simulink model "absSimulation"  (R2013b)
settings: Solver=ode3  StartTime=0.0  StopTime=60  FixedStep=0.0001  MaxStep=0.01  RelTol=1e-3
InitFcn:
  | initAbsSim
StartFcn:
  | initAbsSim
values from neighbouring files (symbols this model uses):
  g = 9.81    [abssim1.mat]    (also in abssim2.mat; abssim3.mat; initAbsSim.m)
  m = 9    [abssim1.mat]    (also in abssim2.mat; abssim3.mat; initAbsSim.m)
  Rd = 0.0625    [abssim1.mat]    (also in abssim2.mat; abssim3.mat; initAbsSim.m)
  tyreData = [0 0.0585778811244 0.114421508325 0.16758915878 0.218139109665 0.266129638158 0.311619021435 0.354665536675 0.395327461053 0.433663071746 0.469730645933 0.503588460789 ... (101 elements, 1x101)]    [abssim1.mat]    (also in abssim2.mat; abssim3.mat; tyreDataGen.m = interp1(x,v,xq, 'spline'))
  v0 = 20    [abssim1.mat]    (also in abssim2.mat; abssim3.mat; initAbsSim.m = 5)
libraries: simulink x2
settings Model: FPTRunName=FPA_Reference  Creator=lasse  LastModifiedBy=Lasse
settings DebuggingCC: SignalRangeChecking=warning
settings HardwareCC: ProdBitPerInt=16  ProdBitPerPointer=8  ProdIntDivRoundTo=Zero  ProdEndianess=LittleEndian  ProdWordSize=8  ProdHWDeviceType=Atmel->AVR
settings ModelReferenceCC: ModelReferenceMinAlgLoopOccurrences=on

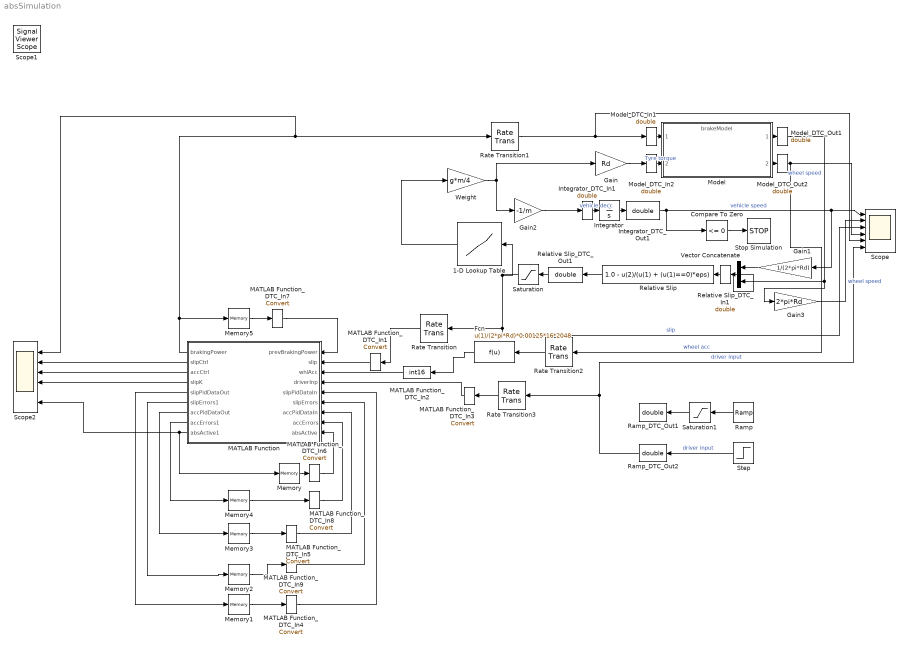
== system absSimulation ==
  1-D Lookup Table : Lookup_n-D  NumberOfTableDimensions=1  BreakpointsForDimension1=[0:100]  Table=tyreData(1:101)  TableDataTypeStr=double  OutDataTypeStr=double  RndMeth=Simplest  InputSameDT=on
  Compare To Zero : simulink/Logic and Bit Operations/Compare To Zero  relop=<=  OutDataTypeStr=boolean
  Fcn : Fcn  Expr=u(1)/(2*pi*Rd)*0.00125*16*2048
  Gain : Gain  Gain=Rd  OutDataTypeStr=double
  Gain1 : Gain  Gain=1/(2*pi*Rd)  OutDataTypeStr=double
  Gain2 : Gain  Gain=-1/m  OutDataTypeStr=double
  Gain3 : Gain  Gain=2*pi*Rd  OutDataTypeStr=double
  Integrator : Integrator  InitialCondition=v0
  Integrator_DTC_In1 : DataTypeConversion  Tag=InsertedToIsolateUnsupportedBlock  OutDataTypeStr=double  LockScale=on
  Integrator_DTC_Out1 : DataTypeConversion  OutDataTypeStr=double
  MATLAB Function : MATLAB Function  TreatAsAtomicUnit=on  SystemSampleTime=0.01
  MATLAB Function_DTC_In{1,3..9} (8 alike) : DataTypeConversion
  MATLAB Function_DTC_In2 : DataTypeConversion  Tag=InsertedToIsolateUnsupportedBlock  OutDataTypeStr=int16  LockScale=on
  Memory : Memory  InheritSampleTime=on
  Memory1 : Memory  X0="[128  100 0 100 0]*2^8"  InheritSampleTime=on
  Memory2 : Memory  X0=[0 0]  InheritSampleTime=on
  Memory3 : Memory  X0=[5 1 0 0 100 0]*2^8  InheritSampleTime=on
  Memory4 : Memory  X0=[0 0]  InheritSampleTime=on
  Memory5 : Memory  InheritSampleTime=on
  Model : ModelReference  ModelNameDialog=brakeModel.slx  SimulationMode=Normal  ModelReferenceVersion=1.18  CopyOfModelName=brakeModel.slx  DefaultDataLogging=on
  Model_DTC_In1 : DataTypeConversion  Tag=InsertedToIsolateUnsupportedBlock  OutDataTypeStr=double  LockScale=on
  Model_DTC_In2 : DataTypeConversion  Tag=InsertedToIsolateUnsupportedBlock  OutDataTypeStr=double  LockScale=on
  Model_DTC_Out1 : DataTypeConversion  OutDataTypeStr=double
  Model_DTC_Out2 : DataTypeConversion  OutDataTypeStr=double
  Ramp : simulink/Sources/Ramp  slope=10  start=0  X0=0
  Ramp_DTC_Out1 : DataTypeConversion  OutDataTypeStr=double
  Ramp_DTC_Out2 : DataTypeConversion  OutDataTypeStr=double
  Rate Transition : RateTransition  OutPortSampleTime=0.01
  Rate Transition1 : RateTransition  OutPortSampleTimeOpt=Inherit  OutPortSampleTime=0.01
  Rate Transition2 : RateTransition  OutPortSampleTime=0.01
  Rate Transition3 : RateTransition  OutPortSampleTime=0.01
  Relative Slip : Fcn  Expr=1.0 - u(2)/(u(1) + (u(1)==0)*eps)
  Relative Slip_DTC_In1 : DataTypeConversion  Tag=InsertedToIsolateUnsupportedBlock  OutDataTypeStr=double  LockScale=on
  Relative Slip_DTC_Out1 : DataTypeConversion  OutDataTypeStr=double
  Saturation : Saturate  UpperLimit=1.0  LowerLimit=0  OutDataTypeStr=double
  Saturation1 : Saturate  UpperLimit=500  LowerLimit=0
  Scope : Scope  NumInputPorts=6
      settings: YMin=19.9955~19.1~0~-17.5~0~475  YMax=20~20~0.045~5~100~525
  Scope2 : Scope  NumInputPorts=6
      settings: YMin=0~19000~-35000~0~-1~0  YMax=100~33000~35000~100~1~1
  Step : Step  After=500  SampleTime=0
  Stop Simulation : Stop
  Vector Concatenate : Concatenate
  Weight : Gain  Gain=g*m/4  OutDataTypeStr=double
  Scope1 : SignalViewerScope  IOType=viewer  RefreshTime=0.035000
  wires:
  Model/1 -> Model_DTC_Out1/1
  Gain1/1 -> Vector Concatenate/1
  Vector Concatenate/1 -> Relative Slip_DTC_In1/1
  Relative Slip/1 -> Relative Slip_DTC_Out1/1
  Weight/1 -> Gain2/1, Gain/1
  Gain/1 -> Model_DTC_In2/1
  Gain2/1 -> Integrator_DTC_In1/1
  Integrator/1 -> Integrator_DTC_Out1/1
  Compare To Zero/1 -> Stop Simulation/1
  Saturation/1 -> Rate Transition/1, Scope/3, 1-D Lookup Table/1  "slip"
  Gain3/1 -> Scope/2  "wheel speed"
  Model/2 -> Model_DTC_Out2/1
  Ramp/1 -> Saturation1/1
  Rate Transition1/1 -> Model_DTC_In1/1, Scope/5
  1-D Lookup Table/1 -> Weight/1
  Ramp_DTC_Out2/1 -> Scope/6, Rate Transition3/1  "driver input"
  Integrator_DTC_Out1/1 -> Scope/1, Gain1/1, Compare To Zero/1  "vehicle speed"
  Relative Slip_DTC_Out1/1 -> Saturation/1
  Relative Slip_DTC_In1/1 -> Relative Slip/1
  Model_DTC_In1/1 -> Model/1
  Model_DTC_In2/1 -> Model/2  "Tyre torque"
  Model_DTC_Out1/1 -> Gain3/1, Vector Concatenate/2  "wheel speed"
  Model_DTC_Out2/1 -> Scope/4, Rate Transition2/1  "wheel acc"
  Rate Transition/1 -> MATLAB Function_DTC_In1/1
  Integrator_DTC_In1/1 -> Integrator/1  "vehicle decc"
  Step/1 -> Ramp_DTC_Out2/1  "driver input"
  Rate Transition2/1 -> Fcn/1
  Fcn/1 -> MATLAB Function_DTC_In2/1
  MATLAB Function_DTC_In2/1 -> MATLAB Function/3(whlAcc)
  Rate Transition3/1 -> MATLAB Function_DTC_In3/1
  MATLAB Function/7(accPidDataOut) -> Memory3/1
  MATLAB Function/9(absActive1) -> Memory/1, Scope2/6
  Memory1/1 -> MATLAB Function_DTC_In4/1
  Memory3/1 -> MATLAB Function_DTC_In5/1
  Memory/1 -> MATLAB Function_DTC_In6/1
  MATLAB Function/2(slipCtrl) -> Scope2/2
  MATLAB Function/3(accCtrl) -> Scope2/3
  MATLAB Function/4(slipK) -> Scope2/4
  MATLAB Function_DTC_In1/1 -> MATLAB Function/2(slip)
  MATLAB Function_DTC_In3/1 -> MATLAB Function/4(driverInp)
  MATLAB Function_DTC_In4/1 -> MATLAB Function/5(slipPidDataIn)
  MATLAB Function_DTC_In5/1 -> MATLAB Function/7(accPidDataIn)
  MATLAB Function_DTC_In6/1 -> MATLAB Function/9(absActive)
  Saturation1/1 -> Ramp_DTC_Out1/1
  MATLAB Function/5(slipPidDataOut) -> Memory1/1
  MATLAB Function/8(accErrors1) -> Memory4/1
  Memory4/1 -> MATLAB Function_DTC_In8/1
  MATLAB Function/6(slipErrors1) -> Memory2/1
  Memory2/1 -> MATLAB Function_DTC_In9/1
  MATLAB Function_DTC_In7/1 -> MATLAB Function/1(prevBrakingPower)
  MATLAB Function_DTC_In8/1 -> MATLAB Function/8(accErrors)
  MATLAB Function_DTC_In9/1 -> MATLAB Function/6(slipErrors)
  Memory5/1 -> MATLAB Function_DTC_In7/1
  MATLAB Function/1(brakingPower) -> Scope2/1, Rate Transition1/1, Memory5/1

== matlab function absSimulation/MATLAB Function ==
  data: prevBrakingPower input; slip input; brakingPower output; slipCtrl output; accCtrl output; slipK output; slipPidDataOut output; slipErrors1 output; whlAcc input; driverInp input; slipPidDataIn input; slipErrors input; accPidDataOut output; accErrors1 output; accPidDataIn input; accErrors input; absActive input; absActive1 output
function [brakingPower, slipCtrl, accCtrl, slipK, slipPidDataOut, slipErrors1, accPidDataOut, accErrors1, absActive1]= fcn(prevBrakingPower, slip,whlAcc,driverInp, slipPidDataIn, slipErrors, accPidDataIn, accErrors, absActive)
% %%%%%%%%%
%     sampleT = 0.00125;
%     PPR = 2048;
%     Rd = 0.0625;
%     desiredSlip = int8(33);
%     
%     desiredAcc = -5;
%     desiredAccInt = int16(desiredAcc/(2*pi*Rd)*sampleT*16*PPR);
%     slipParamsPID = [20 10 0 0.01, prevBrakingPower];
%     accParamsPID = [1 0.5 0 0.01 prevBrakingPower];
%     
%     if abs(whlAcc) > 1000
%         slipK = int8(0);
%     elseif abs(whlAcc) < 10
%         slipK = int8(100);
%     else
%         slipK = int8(100) - int8(abs(whlAcc)/1000);
%     end
% 
%     [slipCtrl, eSlip] = PID(slip, desiredSlip, slipErrors, slipParamsPID);
%     [accCtrl, eAcc] = PID(-whlAcc, desiredAccInt, accErrors, accParamsPID);
% 
%     slipErrors1 = [eSlip slipErrors(1)];
%     accErrors1 = [eAcc accErrors(1)];
%     if absActive
%         brakingPower = prevBrakingPower + slipK*int8(slipCtrl) + (int8(100)-slipK)*int8(accCtrl);
%         absActive1 = absActive;
%     else
%         brakingPower = int8(driverInp);
%         if whlAcc < desiredAcc || slip > desiredSlip
%             absActive1 = 1;
%         else
%             absActive1 = 0;
%         end
%     end
%     
%     brakingPower = checkSaturation(brakingPower, int8([0 100])); 
% %%%    

    sampleT = 0.00125;
    PPR = 2048;
    Rd = 0.0625;
    desiredSlip = int16(33);
    slipPercent = int16(slip*100);
    desiredAcc = -5;
    desiredAccInt = int16(desiredAcc/(2*pi*Rd)*sampleT*16*PPR);
    slipPidData = int16(slipPidDataIn);
    [slipCtrl, slipPidDataOut] = PID(slipPidData, desiredSlip - slipPercent, slipErrors);
    [accCtrl, accPidDataOut] = PID(accPidDataIn, desiredAccInt - whlAcc, accErrors);
    if abs(whlAcc) > 1000
        slipK = int16(0);
    elseif abs(whlAcc) < 10
        slipK = int16(100);
    else
        slipK = int16(100) - int16(abs(whlAcc)/10);
    end
    
    slipErrors1 = [desiredSlip - slipPercent slipErrors(1)];
    accErrors1 = [desiredAccInt - whlAcc accErrors(1)];
    if absActive
        brakingPower = prevBrakingPower + (slipK*int16(slipCtrl)/100 + (int16(100)-slipK)*int16(-accCtrl)/100)*2^-8;
        absActive1 = absActive;
    else
        brakingPower = int16(driverInp);
        if whlAcc < desiredAccInt || slipPercent > desiredSlip
            slipPidDataOut(end) = 0;
            accPidDataOut(end) = 0;
            absActive1 = 1;
        else
            absActive1 = 0;
        end
    end
    
    if brakingPower > slipPidData(5)*2^-8
        brakingPower = slipPidData(5)*2^-8;
    elseif brakingPower < slipPidData(4)*2^-8
        brakingPower = slipPidData(4)*2^-8;
    end
end
% 
% function [ctrl, pidData] = PID(pid, error)
% 
%     K = pid(1);
%     Ti = pid(2);
%     Td = pid(3);
%     tiCtrl = int16(0);
%     
%     pCtrl = int16(K*error);
%     tdCtrl = int16(Td*(error-pid(6)));
%     if pid(6) + error > pid(5) && Ti
%         tiCtrl = int16(pid(5));
%         pidData = int16([K Ti Td pid(4) pid(5) pid(6)]);
%     elseif pid(6) + error < pid(4) && Ti
%         tiCtrl = int16(pid(4));
%         pidData = int16([K Ti Td pid(4) pid(5) pid(6)]);
%     else
%         if Ti
%             tiCtrl = int16(Ti*(pid(6) + error));
%         end
%         pidData = int16([K Ti Td pid(4) pid(5) pid(6)+error]);
%     end
%     
%     if pCtrl + tiCtrl + tdCtrl > pid(5)
%         ctrl = int16(pid(5)*2^-8);
%     else
%         ctrl = int16((pCtrl + tiCtrl + tdCtrl)*2^-8);
%     end
% end

function [ctrl, pidData] = PID(pid, error, prevErrors)
    K = pid(1);
    Ti = pid(2);
    Td = pid(3);
    
    pCtrl = K*(error-prevErrors(1));
    tdCtrl = Td * (error - 2*prevErrors(1) + prevErrors(2));
    tiCtrl = Ti * prevErrors(1);
    
    ctrl = (pCtrl + tdCtrl + tiCtrl);
    pidData = pid;
end
